simulink model "bimbam"  (R2023a)
settings: Solver=VariableStepAuto  StartTime=0.0  StopTime=0.1  RelTol=1e-3
libraries: instrumentseriallib x2
settings Model: Creator=root  LastModifiedBy=root

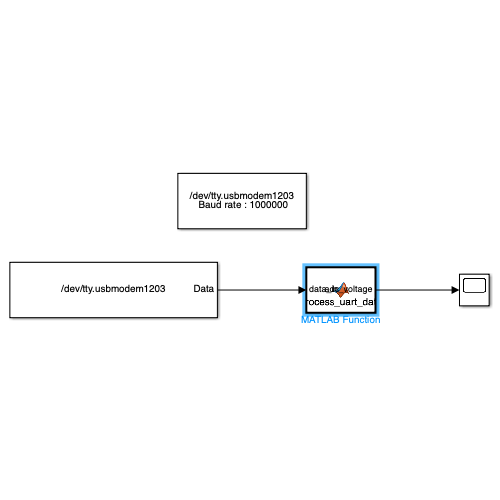
[thumbnail: Simulink's stored preview of the top-level diagram]
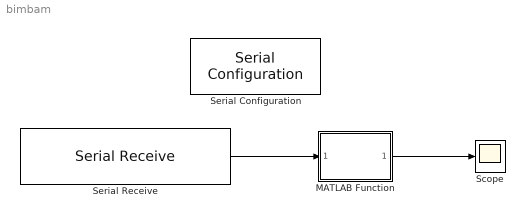
== system bimbam ==
  MATLAB Function : MATLAB Function  TreatAsAtomicUnit=on
  Scope : Scope
  Serial Configuration : instrumentseriallib/Serial Configuration  Priority=-200000  PortSel=/dev/tty.usbmodem1203  Port=/dev/tty.usbmodem1203  ComPort=/dev/tty.usbmodem1203  BaudRate=1000000  DataBits=8  Parity=none  StopBits=1  ByteOrder=little-endian  FlowControl=none  Timeout=10  SimulateUsing=Interpreted execution  BlockInModel=on  aMode=1
  Serial Receive : instrumentseriallib/Serial Receive  Priority=1  PortSel=/dev/tty.usbmodem1203  Port=/dev/tty.usbmodem1203  ComPort=/dev/tty.usbmodem1203  DataType=uint8  SaveDataType=uint8  ToggleHeader=off  Header=[]  ToggleTerminator=off  Terminator=<none>  CustomTerminator=[]  InputFormat=Column major  ToggleDataSize=on  DataSize=[2 2]  EnableBlockingMode=on  ActionDataUnavailable=Output last received value  ActionWhenDataUnavailable=Output last received value  CustomValue=0  SampleTime=0.001  SimulateUsing=Interpreted execution  BlockInModel=on  aMode=1
  wires:
  Serial Receive/1 -> MATLAB Function/1(data_in)
  MATLAB Function/1(adc_voltage) -> Scope/1

== matlab function bimbam/MATLAB Function ==
  data: data_in input; adc_voltage output
function adc_voltage = process_uart_data(data_in)
% Function to process UART data and reconstruct ADC voltage values
% Inputs:
%   data_in - vector of uint8 bytes received from UART
% Output:
%   adc_voltage - scalar double value of ADC voltage in mV

% Persistent buffer to store incoming bytes
persistent buffer;
if isempty(buffer)
    buffer = uint8([]);
end

% Append new data to buffer
buffer = [buffer; data_in(:)];
adc_voltage = NaN; % default output, NaN indicates no valid data

% Process buffer
while length(buffer) >= 4
    if buffer(3) == 170 && buffer(4) == 187 % Check for 0xAA 0xBB
        % Extract data bytes
        high_byte = buffer(1);
        low_byte = buffer(2);
        % Reconstruct adc_value_mv
        adc_value_mv = double(bitshift(uint16(high_byte),8)) + double(low_byte);
        % Output the value
        adc_voltage = adc_value_mv;
        % Remove processed bytes from buffer
        buffer(1:4) = [];
        % Exit function after processing one packet
        return;
    else
        % Remove first byte from buffer and continue
        buffer(1) = [];
    end
end
end
